simulink model "XOR_FanIn3_with2"  (R2024a)
settings: Solver=ode45  StartTime=0.0  StopTime=10.0  RelTol=1e-3  EnableMultiTasking=on
settings Model: Creator=nunkesser  LastModifiedBy=nunkesser
settings SolverCC: AlgebraicLoopSolver=TrustRegion
settings DataIOCC: LimitDataPoints=on  SaveFormat=Array  ReturnWorkspaceOutputs=off
settings OptimizationCC: LifeSpan=inf
settings DebuggingCC: SolverPrmCheckMsg=warning  UnconnectedInputMsg=warning  UnconnectedOutputMsg=warning  UnconnectedLineMsg=warning  SFUnexpectedBacktrackingDiag=warning  SFNoUnconditionalDefaultTransitionDiag=warning  SFExecutionAtInitializationDiag=none  ArithmeticOperatorsInVariantConditions=warning
settings HardwareCC: ProdBitPerPointer=32  ProdBitPerSizeT=32  ProdBitPerPtrDiffT=32  ProdLargestAtomicFloat=None  ProdIntDivRoundTo=Undefined  ProdEndianess=Unspecified  ProdWordSize=32  ProdHWDeviceType=32-bit Generic
settings ModelReferenceCC: PropagateSignalLabelsOutOfModel=off
settings SFSimCC: SimUseLocalCustomCode=off  CustomCodeUndefinedFunction=UseInterfaceOnly
settings RTWCC: RTWUseLocalCustomCode=off  GPUComputeCapability=3.5
settings CodeAppCC: StateflowObjectComments=on
settings GRTTargetCC: TargetLangStandard=C89/C90 (ANSI)
settings ConfigComp: CovMetricSettings=dw  CovSaveCumulativeToWorkspaceVar=on  CovSaveSingleToWorkspaceVar=on  CovExternalEMLEnable=off  CovSFcnEnable=off

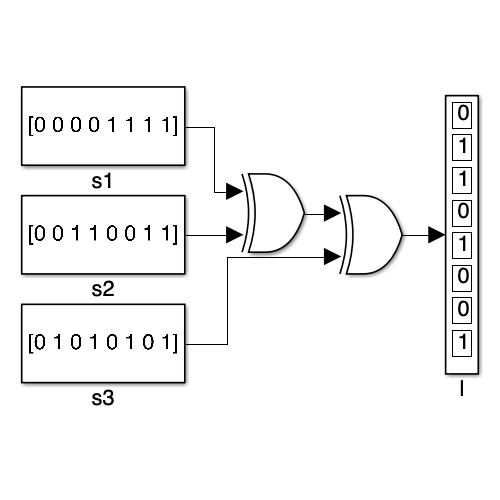
[thumbnail: Simulink's stored preview of the top-level diagram]
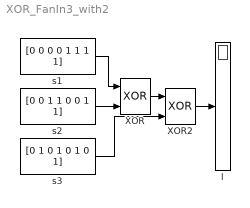
== system XOR_FanIn3_with2 ==
  XOR : Logic  Operator=XOR  IconShape=distinctive  OutDataTypeStr=boolean
  XOR2 : Logic  Operator=XOR  IconShape=distinctive  OutDataTypeStr=boolean
  l : Display
  s1 : Constant  Value=[0 0 0 0 1 1 1 1]  VectorParams1D=off  OutDataTypeStr=boolean
  s2 : Constant  Value=[0 0 1 1 0 0 1 1]  OutDataTypeStr=boolean
  s3 : Constant  Value=[0 1 0 1 0 1 0 1]  OutDataTypeStr=boolean
  wires:
  s1/1 -> XOR/1
  s2/1 -> XOR/2
  XOR/1 -> XOR2/1
  s3/1 -> XOR2/2
  XOR2/1 -> l/1
